simulink model "model"  (R2015a)
settings: Solver=ode45  StartTime=0.0  StopTime=20  RelTol=1e-3
values from neighbouring files (symbols this model uses):
  A = [3.29698189006 1 0 0 -4.20791026518 0 1 0 2.48348543348 0 0 1 ... (16 elements, 4x4)]    [end_of_class.mat]    (also in log_observer_test.mat; parameters.mat)
  B = [1 0 0 0]    [end_of_class.mat]    (also in log_observer_test.mat; parameters.mat)
  C = [-0.0495309545297 0.081302844811 0.0308276179144 0]    [end_of_class.mat]    (also in log_observer_test.mat; parameters.mat)
  K = dlqr(A, B, Q, R)    [compute_gain.m]    (also in end_of_class.mat = [0.679089360081 -1.41789247675 1.07430486636 -0.291654825833; log_observer_test.mat = [0.679089360081 -1.41789247675 1.07430486636 -0.291654825833)
  M = dlqe(A, eye(4), C, eye(4), 1)    [compute_gain.m]    (also in end_of_class.mat = [46.1937797554 31.7894394899 18.6722805315 9.22195693924]; log_observer_test.mat = [13.0934534825 11.0057014889 8.5354108434 5.97963050629])
  Nbar = Nu+K*Nx    [compute_gain.m]    (also in end_of_class.mat = 0.700435596375; log_observer_test.mat = 0.700435596375)
  T = 0.02    [end_of_class.mat]    (also in gera_signals.m; log_observer_test.mat)
settings Model: Creator=Paul  LastModifiedBy=Paul

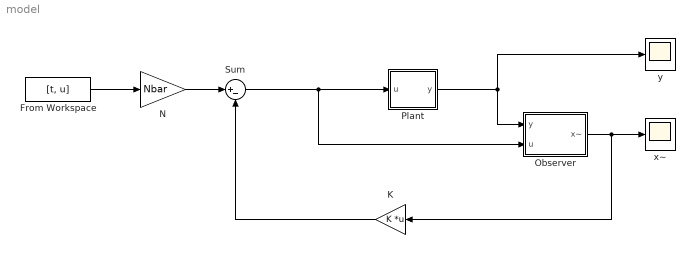
== system model ==
  From Workspace : FromWorkspace  VariableName=[t, u]  SampleTime=T
  K : Gain  Gain=K  Multiplication=Matrix(K*u)
  N : Gain  Gain=Nbar
  Observer : Subsystem
  Plant : Subsystem
  Sum : Sum  Inputs=|+-
  x~ : Scope
      settings: TimeRange=20  YMin=-1000  YMax=0
  y : Scope
      settings: TimeRange=20  YMin=-1000  YMax=0
  wires:
  Plant/1(y) -> Observer/1(y), y/1
  Observer/1(x~) -> K/1, x~/1
  Sum/1 -> Observer/2(u), Plant/1(u)
  N/1 -> Sum/1
  From Workspace/1 -> N/1
  K/1 -> Sum/2

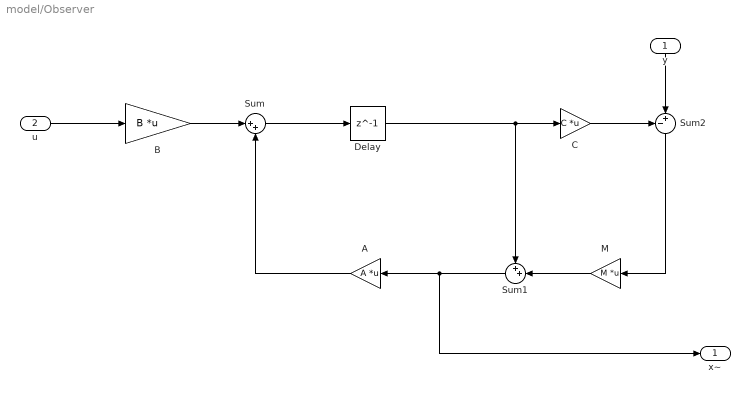
== system model/Observer ==
  y : Inport  PortDimensions=1
  u : Inport  Port=2
  A : Gain  Gain=A  Multiplication=Matrix(K*u)
  B : Gain  Gain=B  Multiplication=Matrix(K*u) (u vector)
  C : Gain  Gain=C  Multiplication=Matrix(K*u)
  Delay : Delay  DelayLength=1  InitialCondition=[0;0;0;0]
  M : Gain  Gain=M  Multiplication=Matrix(K*u) (u vector)
  Sum : Sum  Inputs=|++
  Sum1 : Sum  Inputs=++|
  Sum2 : Sum  Inputs=-+|
  x~ : Outport  PortDimensions=[4,1]
  wires:
  Sum/1 -> Delay/1
  C/1 -> Sum2/1
  Sum2/1 -> M/1
  Delay/1 -> C/1, Sum1/1
  M/1 -> Sum1/2
  A/1 -> Sum/2
  y/1 -> Sum2/2
  u/1 -> B/1
  Sum1/1 -> x~/1, A/1
  B/1 -> Sum/1

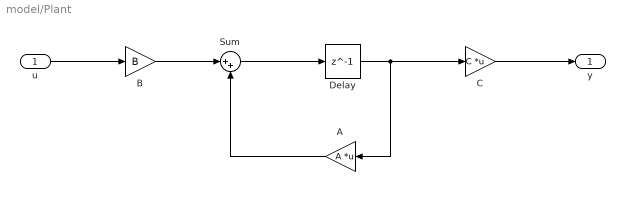
== system model/Plant ==
  u : Inport
  A : Gain  Gain=A  Multiplication=Matrix(K*u)
  B : Gain  Gain=B
  C : Gain  Gain=C  Multiplication=Matrix(K*u)
  Delay : Delay  DelayLength=1  InitialCondition=[0;0;0;0]
  Sum : Sum  Inputs=|++
  y : Outport
  wires:
  u/1 -> B/1
  C/1 -> y/1
  Delay/1 -> A/1, C/1
  B/1 -> Sum/1
  Sum/1 -> Delay/1
  A/1 -> Sum/2
